simulink model "MHI_checked_logic"  (R2018b)
settings: Solver=ode3  StartTime=0.0  StopTime=15000  FixedStep=1  RelTol=1e-3
settings Model: Creator=wcuser7  LastModifiedBy=wcuser7
settings DataIOCC: SaveFormat=StructureWithTime
settings OptimizationCC: LifeSpan=inf
settings DebuggingCC: FcnCallInpInsideContextMsg=warning  LibraryContextMissingDiagnostic=none  SFExecutionAtInitializationDiag=none
settings HardwareCC: ProdBitPerSizeT=32  ProdBitPerPtrDiffT=32  ProdWordSize=32  ProdHWDeviceType=Specified
settings ModelReferenceCC: ModelReferenceNumInstancesAllowed=Single  PropagateSignalLabelsOutOfModel=off
settings CodeAppCC: StateflowObjectComments=on
settings GRTTargetCC: CombineOutputUpdateFcns=off  GRTInterface=on

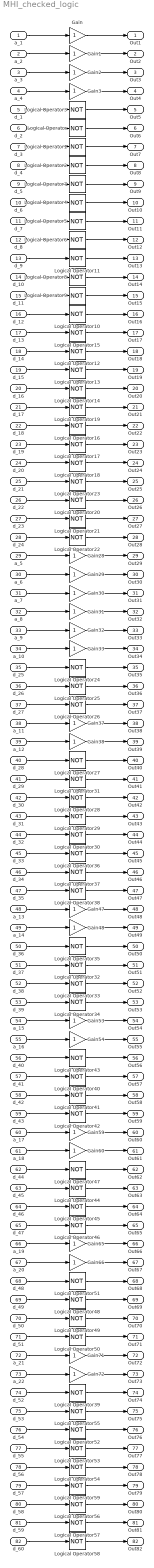
== system MHI_checked_logic ==
  a_1 : Inport  OutDataTypeStr=double
  a_2 : Inport  Port=2  OutDataTypeStr=double
  a_3 : Inport  Port=3  OutDataTypeStr=double
  a_4 : Inport  Port=4  OutDataTypeStr=double
  d_1 : Inport  Port=5  OutDataTypeStr=boolean
  d_2 : Inport  Port=6  OutDataTypeStr=boolean
  d_3 : Inport  Port=7  OutDataTypeStr=boolean
  d_4 : Inport  Port=8  OutDataTypeStr=boolean
  d_5 : Inport  Port=9  OutDataTypeStr=boolean
  d_6 : Inport  Port=10  OutDataTypeStr=boolean
  d_7 : Inport  Port=11  OutDataTypeStr=boolean
  d_8 : Inport  Port=12  OutDataTypeStr=boolean
  d_9 : Inport  Port=13  OutDataTypeStr=boolean
  d_10 : Inport  Port=14  OutDataTypeStr=boolean
  d_11 : Inport  Port=15  OutDataTypeStr=boolean
  d_12 : Inport  Port=16  OutDataTypeStr=boolean
  d_13 : Inport  Port=17  OutDataTypeStr=boolean
  d_14 : Inport  Port=18  OutDataTypeStr=boolean
  d_15 : Inport  Port=19  OutDataTypeStr=boolean
  d_16 : Inport  Port=20  OutDataTypeStr=boolean
  d_17 : Inport  Port=21  OutDataTypeStr=boolean
  d_18 : Inport  Port=22  OutDataTypeStr=boolean
  d_19 : Inport  Port=23  OutDataTypeStr=boolean
  d_20 : Inport  Port=24  OutDataTypeStr=boolean
  d_21 : Inport  Port=25  OutDataTypeStr=boolean
  d_22 : Inport  Port=26  OutDataTypeStr=boolean
  d_23 : Inport  Port=27  OutDataTypeStr=boolean
  d_24 : Inport  Port=28  OutDataTypeStr=boolean
  a_5 : Inport  Port=29  OutDataTypeStr=double
  a_6 : Inport  Port=30  OutDataTypeStr=double
  a_7 : Inport  Port=31  OutDataTypeStr=double
  a_8 : Inport  Port=32  OutDataTypeStr=double
  a_9 : Inport  Port=33  OutDataTypeStr=double
  a_10 : Inport  Port=34  OutDataTypeStr=double
  d_25 : Inport  Port=35  OutDataTypeStr=boolean
  d_26 : Inport  Port=36  OutDataTypeStr=boolean
  d_27 : Inport  Port=37  OutDataTypeStr=boolean
  a_11 : Inport  Port=38  OutDataTypeStr=double
  a_12 : Inport  Port=39  OutDataTypeStr=double
  d_28 : Inport  Port=40  OutDataTypeStr=boolean
  d_29 : Inport  Port=41  OutDataTypeStr=boolean
  d_30 : Inport  Port=42  OutDataTypeStr=boolean
  d_31 : Inport  Port=43  OutDataTypeStr=boolean
  d_32 : Inport  Port=44  OutDataTypeStr=boolean
  d_33 : Inport  Port=45  OutDataTypeStr=boolean
  d_34 : Inport  Port=46  OutDataTypeStr=boolean
  d_35 : Inport  Port=47  OutDataTypeStr=boolean
  a_13 : Inport  Port=48  OutDataTypeStr=double
  a_14 : Inport  Port=49  OutDataTypeStr=double
  d_36 : Inport  Port=50  OutDataTypeStr=boolean
  d_37 : Inport  Port=51  OutDataTypeStr=boolean
  d_38 : Inport  Port=52  OutDataTypeStr=boolean
  d_39 : Inport  Port=53  OutDataTypeStr=boolean
  a_15 : Inport  Port=54  OutDataTypeStr=double
  a_16 : Inport  Port=55  OutDataTypeStr=double
  d_40 : Inport  Port=56  OutDataTypeStr=boolean
  d_41 : Inport  Port=57  OutDataTypeStr=boolean
  d_42 : Inport  Port=58  OutDataTypeStr=boolean
  d_43 : Inport  Port=59  OutDataTypeStr=boolean
  a_17 : Inport  Port=60  OutDataTypeStr=double
  a_18 : Inport  Port=61  OutDataTypeStr=double
  d_44 : Inport  Port=62  OutDataTypeStr=boolean
  d_45 : Inport  Port=63  OutDataTypeStr=boolean
  d_46 : Inport  Port=64  OutDataTypeStr=boolean
  d_47 : Inport  Port=65  OutDataTypeStr=boolean
  a_19 : Inport  Port=66  OutDataTypeStr=double
  a_20 : Inport  Port=67  OutDataTypeStr=double
  d_48 : Inport  Port=68  OutDataTypeStr=boolean
  d_49 : Inport  Port=69  OutDataTypeStr=boolean
  d_50 : Inport  Port=70  OutDataTypeStr=boolean
  d_51 : Inport  Port=71  OutDataTypeStr=boolean
  a_21 : Inport  Port=72  OutDataTypeStr=double
  a_22 : Inport  Port=73  OutDataTypeStr=double
  d_52 : Inport  Port=74  OutDataTypeStr=boolean
  d_53 : Inport  Port=75  OutDataTypeStr=boolean
  d_54 : Inport  Port=76  OutDataTypeStr=boolean
  d_55 : Inport  Port=77  OutDataTypeStr=boolean
  d_56 : Inport  Port=78  OutDataTypeStr=boolean
  d_57 : Inport  Port=79  OutDataTypeStr=boolean
  d_58 : Inport  Port=80  OutDataTypeStr=boolean
  d_59 : Inport  Port=81  OutDataTypeStr=boolean
  d_60 : Inport  Port=82  OutDataTypeStr=boolean
  Gain{,1..3,28..33,37..38,47..48,53..54,59..60,65..66,71..72} (22 alike) : Gain
  Logical Operator{,1..59} (60 alike) : Logic  Operator=NOT  AllPortsSameDT=off  OutDataTypeStr=boolean
  Out1 : Outport
  Out2 : Outport  Port=2
  Out3 : Outport  Port=3
  Out4 : Outport  Port=4
  Out5 : Outport  Port=5
  Out6 : Outport  Port=6
  Out7 : Outport  Port=7
  Out8 : Outport  Port=8
  Out9 : Outport  Port=9
  Out10 : Outport  Port=10
  Out11 : Outport  Port=11
  Out12 : Outport  Port=12
  Out13 : Outport  Port=13
  Out14 : Outport  Port=14
  Out15 : Outport  Port=15
  Out16 : Outport  Port=16
  Out17 : Outport  Port=17
  Out18 : Outport  Port=18
  Out19 : Outport  Port=19
  Out20 : Outport  Port=20
  Out21 : Outport  Port=21
  Out22 : Outport  Port=22
  Out23 : Outport  Port=23
  Out24 : Outport  Port=24
  Out25 : Outport  Port=25
  Out26 : Outport  Port=26
  Out27 : Outport  Port=27
  Out28 : Outport  Port=28
  Out29 : Outport  Port=29
  Out30 : Outport  Port=30
  Out31 : Outport  Port=31
  Out32 : Outport  Port=32
  Out33 : Outport  Port=33
  Out34 : Outport  Port=34
  Out35 : Outport  Port=35
  Out36 : Outport  Port=36
  Out37 : Outport  Port=37
  Out38 : Outport  Port=38
  Out39 : Outport  Port=39
  Out40 : Outport  Port=40
  Out41 : Outport  Port=41
  Out42 : Outport  Port=42
  Out43 : Outport  Port=43
  Out44 : Outport  Port=44
  Out45 : Outport  Port=45
  Out46 : Outport  Port=46
  Out47 : Outport  Port=47
  Out48 : Outport  Port=48
  Out49 : Outport  Port=49
  Out50 : Outport  Port=50
  Out51 : Outport  Port=51
  Out52 : Outport  Port=52
  Out53 : Outport  Port=53
  Out54 : Outport  Port=54
  Out55 : Outport  Port=55
  Out56 : Outport  Port=56
  Out57 : Outport  Port=57
  Out58 : Outport  Port=58
  Out59 : Outport  Port=59
  Out60 : Outport  Port=60
  Out61 : Outport  Port=61
  Out62 : Outport  Port=62
  Out63 : Outport  Port=63
  Out64 : Outport  Port=64
  Out65 : Outport  Port=65
  Out66 : Outport  Port=66
  Out67 : Outport  Port=67
  Out68 : Outport  Port=68
  Out69 : Outport  Port=69
  Out70 : Outport  Port=70
  Out71 : Outport  Port=71
  Out72 : Outport  Port=72
  Out73 : Outport  Port=73
  Out74 : Outport  Port=74
  Out75 : Outport  Port=75
  Out76 : Outport  Port=76
  Out77 : Outport  Port=77
  Out78 : Outport  Port=78
  Out79 : Outport  Port=79
  Out80 : Outport  Port=80
  Out81 : Outport  Port=81
  Out82 : Outport  Port=82
  wires:
  a_1/1 -> Gain/1
  Gain/1 -> Out1/1
  Gain1/1 -> Out2/1
  a_2/1 -> Gain1/1
  a_3/1 -> Gain2/1
  Gain2/1 -> Out3/1
  a_4/1 -> Gain3/1
  Gain3/1 -> Out4/1
  Logical Operator/1 -> Out6/1
  d_2/1 -> Logical Operator/1
  Logical Operator1/1 -> Out7/1
  Logical Operator2/1 -> Out8/1
  d_4/1 -> Logical Operator2/1
  d_3/1 -> Logical Operator1/1
  d_7/1 -> Logical Operator5/1
  d_8/1 -> Logical Operator6/1
  Logical Operator7/1 -> Out9/1
  Logical Operator6/1 -> Out12/1
  Logical Operator4/1 -> Out10/1
  d_6/1 -> Logical Operator4/1
  Logical Operator5/1 -> Out11/1
  d_5/1 -> Logical Operator7/1
  d_11/1 -> Logical Operator9/1
  d_12/1 -> Logical Operator10/1
  Logical Operator11/1 -> Out13/1
  Logical Operator10/1 -> Out16/1
  Logical Operator8/1 -> Out14/1
  d_10/1 -> Logical Operator8/1
  Logical Operator9/1 -> Out15/1
  d_9/1 -> Logical Operator11/1
  d_15/1 -> Logical Operator13/1
  d_16/1 -> Logical Operator14/1
  Logical Operator15/1 -> Out17/1
  Logical Operator14/1 -> Out20/1
  Logical Operator12/1 -> Out18/1
  d_14/1 -> Logical Operator12/1
  Logical Operator13/1 -> Out19/1
  d_13/1 -> Logical Operator15/1
  d_19/1 -> Logical Operator17/1
  d_20/1 -> Logical Operator18/1
  Logical Operator19/1 -> Out21/1
  Logical Operator18/1 -> Out24/1
  Logical Operator16/1 -> Out22/1
  d_18/1 -> Logical Operator16/1
  Logical Operator17/1 -> Out23/1
  d_17/1 -> Logical Operator19/1
  d_23/1 -> Logical Operator21/1
  d_24/1 -> Logical Operator22/1
  Logical Operator23/1 -> Out25/1
  Logical Operator22/1 -> Out28/1
  Logical Operator20/1 -> Out26/1
  d_22/1 -> Logical Operator20/1
  Logical Operator21/1 -> Out27/1
  d_21/1 -> Logical Operator23/1
  a_6/1 -> Gain29/1
  Gain29/1 -> Out30/1
  Gain28/1 -> Out29/1
  a_5/1 -> Gain28/1
  Gain31/1 -> Out32/1
  a_8/1 -> Gain31/1
  Gain30/1 -> Out31/1
  a_7/1 -> Gain30/1
  Gain33/1 -> Out34/1
  a_10/1 -> Gain33/1
  Gain32/1 -> Out33/1
  a_9/1 -> Gain32/1
  d_27/1 -> Logical Operator26/1
  d_26/1 -> Logical Operator25/1
  d_25/1 -> Logical Operator24/1
  Logical Operator25/1 -> Out36/1
  Logical Operator24/1 -> Out35/1
  Logical Operator26/1 -> Out37/1
  Gain38/1 -> Out39/1
  a_11/1 -> Gain37/1
  Gain37/1 -> Out38/1
  a_12/1 -> Gain38/1
  Logical Operator27/1 -> Out40/1
  Logical Operator31/1 -> Out41/1
  d_28/1 -> Logical Operator27/1
  d_29/1 -> Logical Operator31/1
  Logical Operator28/1 -> Out42/1
  Logical Operator29/1 -> Out43/1
  d_30/1 -> Logical Operator28/1
  d_31/1 -> Logical Operator29/1
  Logical Operator30/1 -> Out44/1
  Logical Operator36/1 -> Out45/1
  d_32/1 -> Logical Operator30/1
  d_33/1 -> Logical Operator36/1
  Logical Operator37/1 -> Out46/1
  Logical Operator38/1 -> Out47/1
  d_34/1 -> Logical Operator37/1
  d_35/1 -> Logical Operator38/1
  Gain47/1 -> Out48/1
  a_14/1 -> Gain48/1
  Gain48/1 -> Out49/1
  a_13/1 -> Gain47/1
  d_38/1 -> Logical Operator33/1
  d_37/1 -> Logical Operator32/1
  Logical Operator32/1 -> Out51/1
  Logical Operator34/1 -> Out53/1
  d_36/1 -> Logical Operator35/1
  Logical Operator33/1 -> Out52/1
  Logical Operator35/1 -> Out50/1
  d_39/1 -> Logical Operator34/1
  a_15/1 -> Gain53/1
  Gain54/1 -> Out55/1
  a_16/1 -> Gain54/1
  Gain53/1 -> Out54/1
  d_43/1 -> Logical Operator42/1
  Logical Operator43/1 -> Out56/1
  Logical Operator41/1 -> Out58/1
  Logical Operator40/1 -> Out57/1
  d_41/1 -> Logical Operator40/1
  a_18/1 -> Gain60/1
  Gain59/1 -> Out60/1
  Gain60/1 -> Out61/1
  d_42/1 -> Logical Operator41/1
  d_40/1 -> Logical Operator43/1
  Logical Operator42/1 -> Out59/1
  a_17/1 -> Gain59/1
  d_47/1 -> Logical Operator46/1
  Logical Operator47/1 -> Out62/1
  Logical Operator45/1 -> Out64/1
  Logical Operator44/1 -> Out63/1
  d_45/1 -> Logical Operator44/1
  a_20/1 -> Gain66/1
  Gain65/1 -> Out66/1
  Gain66/1 -> Out67/1
  d_46/1 -> Logical Operator45/1
  d_44/1 -> Logical Operator47/1
  Logical Operator46/1 -> Out65/1
  a_19/1 -> Gain65/1
  d_51/1 -> Logical Operator50/1
  Logical Operator51/1 -> Out68/1
  Logical Operator49/1 -> Out70/1
  Logical Operator48/1 -> Out69/1
  d_49/1 -> Logical Operator48/1
  a_22/1 -> Gain72/1
  Gain71/1 -> Out72/1
  Gain72/1 -> Out73/1
  d_50/1 -> Logical Operator49/1
  d_48/1 -> Logical Operator51/1
  Logical Operator50/1 -> Out71/1
  a_21/1 -> Gain71/1
  Logical Operator53/1 -> Out77/1
  d_52/1 -> Logical Operator39/1
  d_54/1 -> Logical Operator52/1
  d_53/1 -> Logical Operator55/1
  Logical Operator39/1 -> Out74/1
  d_55/1 -> Logical Operator53/1
  Logical Operator52/1 -> Out76/1
  Logical Operator55/1 -> Out75/1
  Logical Operator57/1 -> Out81/1
  d_56/1 -> Logical Operator54/1
  d_58/1 -> Logical Operator56/1
  d_57/1 -> Logical Operator59/1
  Logical Operator54/1 -> Out78/1
  d_59/1 -> Logical Operator57/1
  Logical Operator56/1 -> Out80/1
  Logical Operator59/1 -> Out79/1
  d_60/1 -> Logical Operator58/1
  Logical Operator58/1 -> Out82/1
  d_1/1 -> Logical Operator3/1
  Logical Operator3/1 -> Out5/1
